simulink model "autosar_composition"  (R2022b)
settings: Solver=FixedStepDiscrete  StartTime=0.0  StopTime=10.0  RelTol=1e-3  EnableMultiTasking=on
model workspace (MATLAB code in the model file):
  | TPSPrimaryPercent_LkupTbl = Simulink.LookupTable;
  | TPSPrimaryPercent_LkupTbl.Table.DataType = 'single';
  | TPSPrimaryPercent_LkupTbl.Table.Min = [];
  | TPSPrimaryPercent_LkupTbl.Table.Max = [];
  | TPSPrimaryPercent_LkupTbl.Table.Unit = '';
  | TPSPrimaryPercent_LkupTbl.Table.FieldName = 'Table';
  | TPSPrimaryPercent_LkupTbl.Table.Description = '';
  | TPSPrimaryPercent_LkupTbl.Table.Value = ...
  |   [0 10 20 30 40 50 60 70 80 90 100];
  | TPSPrimaryPercent_LkupTbl.BreakpointsSpecification = 'Explicit values';
  | TPSPrimaryPercent_LkupTbl.SupportTunableSize = false;
  | TPSPrimaryPercent_LkupTbl.Breakpoints.DataType = 'single';
  | TPSPrimaryPercent_LkupTbl.Breakpoints.Min = [];
  | TPSPrimaryPercent_LkupTbl.Breakpoints.Max = [];
  | TPSPrimaryPercent_LkupTbl.Breakpoints.Unit = '';
  | TPSPrimaryPercent_LkupTbl.Breakpoints.FieldName = 'BP1';
  | TPSPrimaryPercent_LkupTbl.Breakpoints.Description = '';
  | TPSPrimaryPercent_LkupTbl.Breakpoints.Value = single(linspace(170, 966, 11));
  | TPSPrimaryPercent_LkupTbl.Breakpoints.TunableSizeName = 'N1';
  | TPSPrimaryPercent_LkupTbl.CoderInfo.StorageClass = 'Auto';
  | TPSPrimaryPercent_LkupTbl.StructTypeInfo.Name = 'MyStruct';
  | TPSPrimaryPercent_LkupTbl.StructTypeInfo.DataScope = 'Auto';
  | TPSPrimaryPercent_LkupTbl.StructTypeInfo.HeaderFileName = '';
  | 
  | TPSSecondaryPercent_LkupTbl = copy(TPSPrimaryPercent_LkupTbl);
  | TPSSecondaryPercent_LkupTbl.Table.Value = ...
  |   [100 90 80 70 60 50 40 30 20 10 0];
settings Model: Creator=The MathWorks, Inc.  LastModifiedBy=The MathWorks, Inc.
settings SolverCC: AlgebraicLoopSolver=TrustRegion  AutoInsertRateTranBlk=on  MaxZcPerStep=1
settings OptimizationCC: DefaultParameterBehavior=Inlined  PassReuseOutputArgsAs=Individual arguments  ZeroExternalMemoryAtStartup=off  ZeroInternalMemoryAtStartup=off  EfficientTunableParamExpr=on
settings DebuggingCC: ParameterTunabilityLossMsg=error  UnconnectedInputMsg=warning  UnconnectedOutputMsg=warning  UnconnectedLineMsg=warning  SFMachineParentedDataDiag=warning  ArithmeticOperatorsInVariantConditions=warning
settings ModelReferenceCC: EnableRefExpFcnMdlSchedulingChecks=on  ModelReferenceNumInstancesAllowed=Single
settings SFSimCC: SimUseLocalCustomCode=off  MATLABDynamicMemAlloc=off  CustomCodeUndefinedFunction=UseInterfaceOnly
settings RTWCC: Description=AUTOSAR  SystemTargetFile=autosar.tlc  GenCodeOnly=on  TemplateMakefile=ert_default_tmf  GenerateReport=on  RTWUseLocalCustomCode=off  IncludeHyperlinkInReport=on  LaunchReport=on  GenerateTraceInfo=on  GenerateTraceReport=on  GenerateTraceReportSl=on  GenerateTraceReportSf=on  GenerateTraceReportEml=on  DLArmComputeVersion=19.05
settings CodeAppCC: ForceParamTrailComments=on  IgnoreCustomStorageClasses=off  OperatorAnnotations=on  SimulinkDataObjDesc=on  SFDataObjDesc=on  InsertBlockDesc=on
settings STFCustomTargetCC: TargetLangStandard=C99 (ISO)  MultiwordLength=256  ParMdlRefBuildCompliant=on  CompOptLevelCompliant=on  IncludeMdlTerminateFcn=off  CombineOutputUpdateFcns=on  SuppressErrorStatus=on  ERTCustomFileBanners=on  SupportNonFinite=off  SupportComplex=off  SupportContinuousTime=off  SupportNonInlinedSFcns=off  RemoveResetFunc=on  MATLABClassNameForMDSCustomization=Simulink.SoftwareTarget.ERTCustomization  CPPClassGenCompliant=on  AutosarCompliant=on  UseToolchainInfoCompliant=on  LookupTableObjectStructAxisOrder=2,1,3,4,...  LUTObjectStructOrderEvenSpacing=Size,Table,Breakpoints  SystemTargetFile=autosar.tlc
settings ERTTargetCC: TargetLangStandard=C99 (ISO)  ConcurrentExecutionCompliant=off  IncludeMdlTerminateFcn=off  SuppressErrorStatus=on  SupportNonFinite=off  SupportComplex=off  ModelStepFunctionPrototypeControlCompliant=off  AutosarCompliant=on  LookupTableObjectStructAxisOrder=2,1,3,4,...  LUTObjectStructOrderEvenSpacing=Size,Table,Breakpoints  InlinedParameterPlacement=NonHierarchical  ERTCustomFileTemplate=example_file_process.tlc

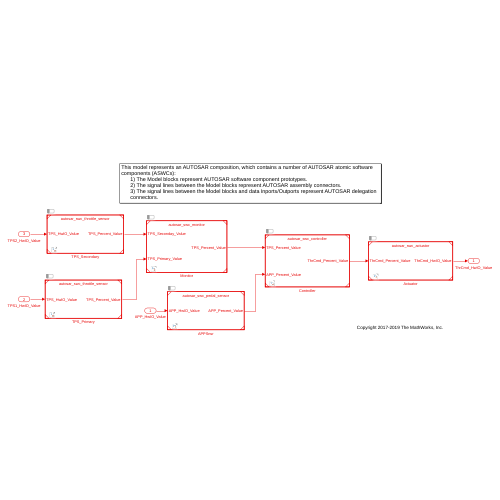
[thumbnail: Simulink's stored preview of the top-level diagram]
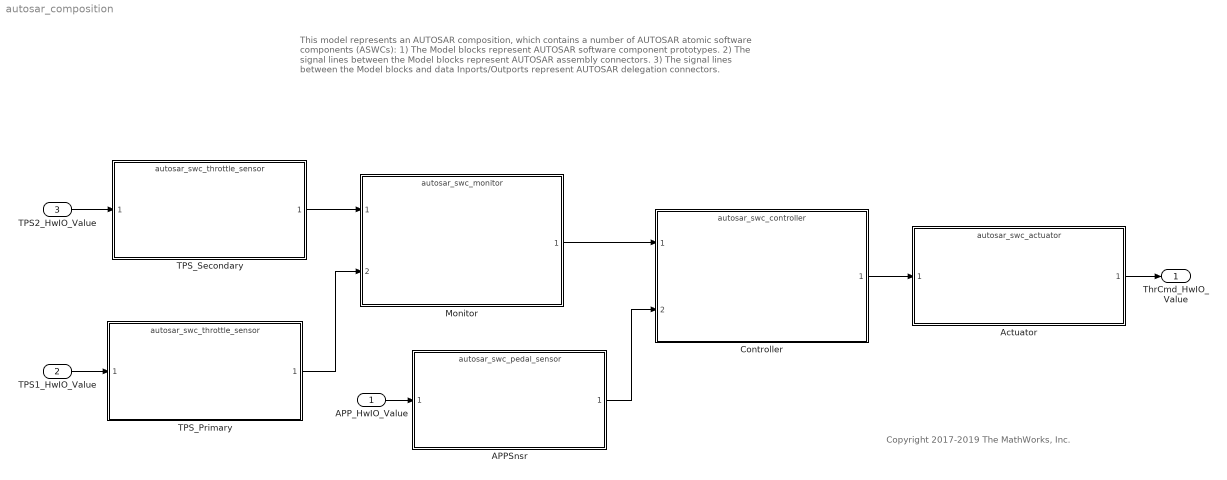
== system autosar_composition ==
  note: This model represents an AUTOSAR composition, which contains a number of AUTOSAR atomic software components (ASWCs):
      | 1) The Model blocks represent AUTOSAR software component prototypes.
      | 2) The signal lines between the Model blocks represent AUTOSAR assembly connectors.
      | 3) The signal lines between the Model blocks and data Inports/Outports represent AUTOSAR delegation connectors.
  note: Copyright 2017-2019 The MathWorks, Inc.
  APP_HwIO_Value : Inport  OutDataTypeStr=uint16  PortDimensions=1
  TPS1_HwIO_Value : Inport  Port=2  OutDataTypeStr=uint16  PortDimensions=1
  TPS2_HwIO_Value : Inport  Port=3  OutDataTypeStr=uint16  PortDimensions=1
  APPSnsr : ModelReference  ModelNameDialog=autosar_swc_pedal_sensor.slx  SimulationMode=Normal  ScheduleRates=on  ScheduleRatesWith=Schedule Editor  PortDiscreteRates=0.005  CachedPortDiscreteRates=[0.005]  ModelReferenceVersion=6.0
  Actuator : ModelReference  ModelNameDialog=autosar_swc_actuator.slx  SimulationMode=Normal  ScheduleRates=on  ScheduleRatesWith=Schedule Editor  PortDiscreteRates=0.005  CachedPortDiscreteRates=[0.005]  ModelReferenceVersion=6.0
  Controller : ModelReference  ModelNameDialog=autosar_swc_controller.slx  SimulationMode=Normal  ScheduleRates=on  ScheduleRatesWith=Schedule Editor  PortDiscreteRates=0.005  CachedPortDiscreteRates=[0.005]  ModelReferenceVersion=7.0
  Monitor : ModelReference  ModelNameDialog=autosar_swc_monitor.slx  SimulationMode=Normal  ScheduleRates=on  ScheduleRatesWith=Schedule Editor  PortDiscreteRates=0.005  CachedPortDiscreteRates=[0.005]  ModelReferenceVersion=7.0
  TPS_Primary : ModelReference  ModelNameDialog=autosar_swc_throttle_sensor.slx  UsingDefaultArgumentValue=0  SimulationMode=Normal  ScheduleRates=on  ScheduleRatesWith=Schedule Editor  PortDiscreteRates=0.005  CachedPortDiscreteRates=[0.005]  ModelReferenceVersion=6.0
  TPS_Secondary : ModelReference  ModelNameDialog=autosar_swc_throttle_sensor.slx  UsingDefaultArgumentValue=0  SimulationMode=Normal  ScheduleRates=on  ScheduleRatesWith=Schedule Editor  PortDiscreteRates=0.005  CachedPortDiscreteRates=[0.005]  ModelReferenceVersion=6.0
  ThrCmd_HwIO_Value : Outport  OutDataTypeStr=int16  PortDimensions=1  VectorParamsAs1DForOutWhenUnconnected=off
  wires:
  APPSnsr/1 -> Controller/2
  Controller/1 -> Actuator/1
  Monitor/1 -> Controller/1
  TPS_Primary/1 -> Monitor/2
  TPS_Secondary/1 -> Monitor/1
  APP_HwIO_Value/1 -> APPSnsr/1
  Actuator/1 -> ThrCmd_HwIO_Value/1
  TPS2_HwIO_Value/1 -> TPS_Secondary/1
  TPS1_HwIO_Value/1 -> TPS_Primary/1
